simulink model "P3_9"  (R2024b)
settings: Solver=VariableStepAuto  StartTime=0.0  StopTime=10.0  RelTol=1e-3
settings Model: Creator=Rj Avro Biswas  LastModifiedBy=Rj Avro Biswas

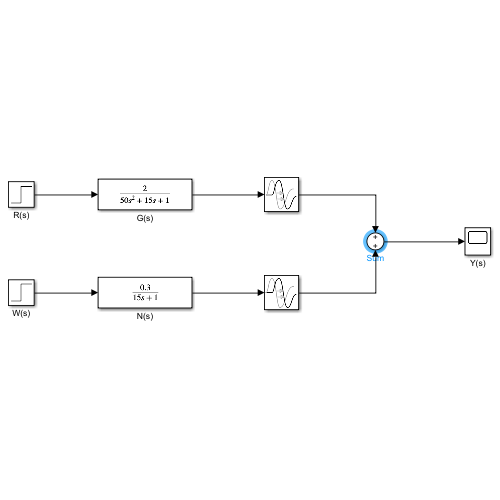
[thumbnail: Simulink's stored preview of the top-level diagram]
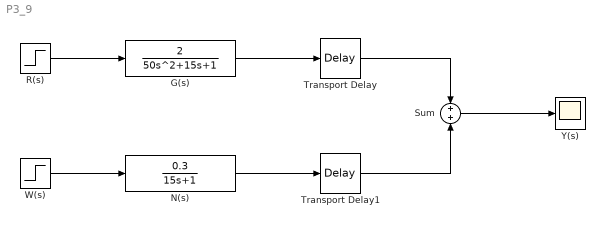
== system P3_9 ==
  G(s) : TransferFcn  Numerator=2  Denominator=[50 15 1]
  N(s) : TransferFcn  Numerator=0.3  Denominator=[15 1]
  R(s) : Step  After=30  SampleTime=0
  Sum : Sum  Inputs=+|+
  Transport Delay : TransportDelay  DelayTime=5
  Transport Delay1 : TransportDelay  DelayTime=5
  W(s) : Step  Time=2  After=20  SampleTime=0
  Y(s) : Scope
  wires:
  G(s)/1 -> Transport Delay/1
  N(s)/1 -> Transport Delay1/1
  Sum/1 -> Y(s)/1
  R(s)/1 -> G(s)/1
  W(s)/1 -> N(s)/1
  Transport Delay/1 -> Sum/1
  Transport Delay1/1 -> Sum/2
